simulink model "test1"  (R2014a)
settings: Solver=ode45  StartTime=0.0  StopTime=10.0  RelTol=1e-3
settings Model: Creator=wang.shiyu  LastModifiedBy=wang.shiyu
settings OptimizationCC: BlockReduction=off  ConditionallyExecuteInputs=off  InlineParams=on
settings DebuggingCC: AlgebraicLoopMsg=error
settings HardwareCC: ProdHWDeviceType=ASIC/FPGA->ASIC/FPGA  ProdEqTarget=off

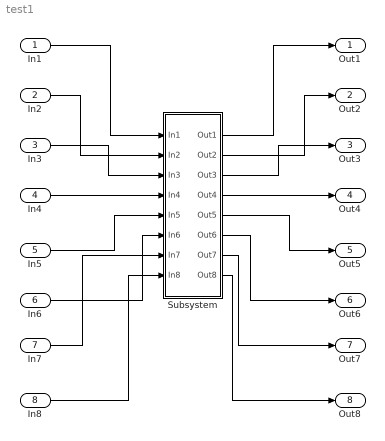
== system test1 ==
  In1 : Inport  OutDataTypeStr=boolean  SampleTime=1
  In2 : Inport  Port=2  OutDataTypeStr=boolean  SampleTime=1
  In3 : Inport  Port=3  OutDataTypeStr=boolean  SampleTime=1
  In4 : Inport  Port=4  OutDataTypeStr=boolean  SampleTime=1
  In5 : Inport  Port=5  OutDataTypeStr=boolean  SampleTime=1
  In6 : Inport  Port=6  OutDataTypeStr=boolean  SampleTime=1
  In7 : Inport  Port=7  OutDataTypeStr=boolean  SampleTime=1
  In8 : Inport  Port=8  OutDataTypeStr=boolean  SampleTime=1
  Subsystem : Subsystem  TreatAsAtomicUnit=on
  Out1 : Outport
  Out2 : Outport  Port=2
  Out3 : Outport  Port=3
  Out4 : Outport  Port=4
  Out5 : Outport  Port=5
  Out6 : Outport  Port=6
  Out7 : Outport  Port=7
  Out8 : Outport  Port=8
  wires:
  In1/1 -> Subsystem/1(In1)
  In2/1 -> Subsystem/2(In2)
  In3/1 -> Subsystem/3(In3)
  In4/1 -> Subsystem/4(In4)
  In5/1 -> Subsystem/5(In5)
  In6/1 -> Subsystem/6(In6)
  In7/1 -> Subsystem/7(In7)
  In8/1 -> Subsystem/8(In8)
  Subsystem/1(Out1) -> Out1/1
  Subsystem/2(Out2) -> Out2/1
  Subsystem/3(Out3) -> Out3/1
  Subsystem/4(Out4) -> Out4/1
  Subsystem/5(Out5) -> Out5/1
  Subsystem/6(Out6) -> Out6/1
  Subsystem/7(Out7) -> Out7/1
  Subsystem/8(Out8) -> Out8/1

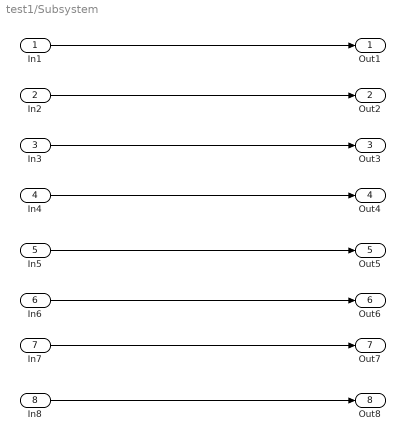
== system test1/Subsystem ==
  In1 : Inport  OutDataTypeStr=boolean  SampleTime=1
  In2 : Inport  Port=2  OutDataTypeStr=boolean  SampleTime=1
  In3 : Inport  Port=3  OutDataTypeStr=boolean  SampleTime=1
  In4 : Inport  Port=4  OutDataTypeStr=boolean  SampleTime=1
  In5 : Inport  Port=5  OutDataTypeStr=boolean  SampleTime=1
  In6 : Inport  Port=6  OutDataTypeStr=boolean  SampleTime=1
  In7 : Inport  Port=7  OutDataTypeStr=boolean  SampleTime=1
  In8 : Inport  Port=8  OutDataTypeStr=boolean  SampleTime=1
  Out1 : Outport
  Out2 : Outport  Port=2
  Out3 : Outport  Port=3
  Out4 : Outport  Port=4
  Out5 : Outport  Port=5
  Out6 : Outport  Port=6
  Out7 : Outport  Port=7
  Out8 : Outport  Port=8
  wires:
  In1/1 -> Out1/1
  In2/1 -> Out2/1
  In3/1 -> Out3/1
  In4/1 -> Out4/1
  In5/1 -> Out5/1
  In6/1 -> Out6/1
  In7/1 -> Out7/1
  In8/1 -> Out8/1
